simulink model "EMC_no_hand"  (R2015a)
settings: Solver=ode4  SolverMode=MultiTasking  StartTime=0.0  StopTime=inf  FixedStep=BKIN_STEP_TIME  RelTol=1e-3
StartFcn:
  |  warndlg('Dexterit-E models cannot run under simulation. Please compile your model and run it from within Dexterit-E.');set_param(bdroot,'SimulationCommand','stop')
model workspace (MAT data in the model file):
  BKIN_KINEMATIC_FRAME_SIZE = 400
  BKIN_STEP_TIME = 0.00025
  COLOR = 4
  COL_X = 1
  COL_Y = 2
  E_NO_EVENT = 0
  LOAD_X = 1
  LOAD_Y = 2
  MOVEMENT_DELAY = 3
  PATH_LENGTH = 1
  PATH_PERIOD = 2
  POST_TRIAL_DELAY = 4
  RADIUS = 3
  TRAJECTORY = 1
  TRAJECTORY_TYPE = 2
  TRIAL_END = 3
  TRIAL_MOVEMENT = 2
  TRIAL_RESET = 4
  TRIAL_START = 1
  X_POSITION = 1
  Y_POSITION = 2
  col_x = 1
  col_y = 2
  ANGULAR_THRESHOLD = 5
  GAZE_EXIT = 6
  START_REACHED = 7
  FIXATION_DURATION = 6
  TRACKING_TARGET_ROW = 7
  FEEDBACK_COLOR = 5
  CROSS_LOGICAL_RADIUS = 8
  DETECT_FIXATION = 8
  GAZE_IN_TARGET = 5
  START_STABILIZATION = 9
  HAND_IN_TARGET = 9
  BACKGROUND_LOAD = 10
  DIST_BETWEEN_TRAJ = 11
  STRAIGHT_PAUSE_TIME = 12
libraries: simulink x14, xpcrtudplib x12, xpcutilitieslib x10, xpcobsoletelib x8, slrtlib x2, ethercat x2, General x2, Video x2
(part 6 of 6)

== matlab function EMC_no_hand/DataLogging/Poll KINARM/createKINData/record errors ==
  data: newMessage output; ECATMessages input; cycle input; step_time input; sentMessageCount output
function [newMessage, sentMessageCount] = fcn(ECATMessages, cycle, step_time)

    persistent lastECATMessages outCount memoryBuffer waitingMsgCount sentCount
    
    if isempty(lastECATMessages)
        lastECATMessages = ECATMessages;
        memoryBuffer = zeros(50, 6);
        waitingMsgCount = 0;
        outCount = 0;
        sentCount = 0;
    end
    
    stepsPerFrame = 0.001 / step_time;

    %copy over the errors from ethercat drives
    for drive=1:4
        if waitingMsgCount >= 50
            continue;
        end
        
        if ECATMessages(drive, 3) ~= lastECATMessages(drive, 3) && ECATMessages(drive, 3) ~= 0
            waitingMsgCount = waitingMsgCount + 1;
%            memoryBuffer(waitingMsgCount,:) = [cycle, ECATMessages(drive,1), ECATMessages(drive,2), ECATMessages(drive,3), ECATMessages(drive, 4), ECATMessages(drive,5)];
            memoryBuffer(waitingMsgCount,1) = cycle;
            memoryBuffer(waitingMsgCount,2:6) = ECATMessages(drive,:);
        end
    end
    
    newMessage = zeros(1,6);
    %if we have an error to send we must send it for a few frames because we only send
    %some frames to the GUI computer. The only safe way to handle this is to count
    %the number of real-time frames vs the frequency we send to the GUI computer on.
    %I wanted to use the actual frame number we send to the GUI, but the trouble is
    %we don't know which of the kinematic frames gets sent to the GUI, it's just one
    %of the 2 or 4 that happens for each frame we send to the GUI. 
    %So instead here I cop out and just count 2 or 4 frames and then send something new.
    if waitingMsgCount > 0
        newMessage = memoryBuffer(1,:);
        outCount = outCount + 1;
        
        %we've sent the frame enough times...
        if outCount >= stepsPerFrame
            %shift the list so the first row is the next thing to send.
            memoryBuffer(1:end-1,:) = memoryBuffer(2:end,:);
            waitingMsgCount = waitingMsgCount - 1;
            sentCount = sentCount + 1;
            outCount = 0;  
            
            %if we still have another frame to send then copy it out..
            if waitingMsgCount > 0
                newMessage = memoryBuffer(1,:);
                outCount = 1;
            end
        end
    end
    
    lastECATMessages = ECATMessages;
    sentMessageCount = sentCount;
end

== matlab function EMC_no_hand/DataLogging/Poll KINARM/make KINData bus/splitKINData arm1 ==
  data: robot_row input; link_lengths output; pointer_offset output; shoulder_loc output; arm_orientation output; shoulder_ang output; elbow_ang output; shoulder_ang_velocity output; elbow_ang_velocity output; shoulder_ang_acceleration output; elbow_ang_acceleration output; joint_torque_cmd output; motor_torque_cmd output; link_angle output; link_velocity output; link_acceleration output; hand_position output; hand_velocity output; hand_acceleration output; elbow_position output; elbow_velocity output; elbow_acceleration output; motor_status output; force_sensor_force_uvw output; force_sensor_torque_uvw output; force_sensor_force_xyz output; force_sensor_torque_xyz output; force_sensor_timestamp output
function [link_lengths, pointer_offset, shoulder_loc, arm_orientation, ...
    shoulder_ang, elbow_ang, shoulder_ang_velocity, elbow_ang_velocity, shoulder_ang_acceleration, elbow_ang_acceleration, ...
    joint_torque_cmd, motor_torque_cmd, ...
    link_angle, link_velocity, link_acceleration, ...
    hand_position, hand_velocity, hand_acceleration, ...
    elbow_position, elbow_velocity, elbow_acceleration, ...
    motor_status, ...
    force_sensor_force_uvw, force_sensor_torque_uvw, force_sensor_force_xyz, force_sensor_torque_xyz, force_sensor_timestamp] = splitKINData(robot_row)

link_lengths = robot_row(1,1:2);                % L1, L2 length in m
pointer_offset = robot_row(1,3);                % perpendicular distance from L2 to subject pointer (m)
shoulder_loc = robot_row(1,4:5);                % shoulder x,y position (m) (global coordinates)
arm_orientation = robot_row(1,6);                % subject's expected arm orientation (1: right, 2: left)
shoulder_ang = robot_row(1,7);				% shoulder joint angle, with correction for offsets (see above) (rad)
elbow_ang = robot_row(1,8);					% elbow joint angle, with correction for offsets (see above) (rad)
shoulder_ang_velocity = robot_row(1,9);             % shoulder joint angular velocity (rad/s)
elbow_ang_velocity = robot_row(1,10);               % elbow joint angular velocity (rad/s)
shoulder_ang_acceleration = robot_row(1,11);        % shoulder joint angular acceleration (rad/s^2)
elbow_ang_acceleration = robot_row(1,12);           % elbow joint angular acceleration (rad/s^2)
joint_torque_cmd = robot_row(1,13:14);          % commanded shoulder (1), and elbow (2) torque (Nm)
motor_torque_cmd = robot_row(1,15:16);          % commanded motor 1 (1) and 2 (2) torque (shoulder torque less elbow torque) (Nm)

link_angle = robot_row(1,17:18);                % upper arm angle with corrections, orientation-independent (see above) (rad)
link_velocity = robot_row(1,19:20);             % upper arm angular velocity, orientation-independent (see above) (rad/s)
link_acceleration = robot_row(1,21:22);         % upper arm angular acceleration, orientation-independent (see above) (rad/s^2)


hand_position = robot_row(1,23:24);             % fingertip position in x,y (m)
hand_velocity = robot_row(1,25:26);             % fingertip velocity in x,y (m/s)
hand_acceleration = robot_row(1,27:28);         % fingertip acceleration in x,y (m/s^2)

elbow_position = robot_row(1,29:30);
elbow_velocity =  robot_row(1,31:32);
elbow_acceleration = robot_row(1,33:34);

% shoulder_velocity_filt = robot_row(1,35);
% elbow_velocity_filt = robot_row(1,36);

motor_status = robot_row(1,37);                 % motor status (bitfield; each 0: motor enabled, 1: motor disabled/faulted)

force_sensor_force_uvw = robot_row(1,38:40);    % force measured by force sensor along u,v,w in its local coordinate system (N)
force_sensor_torque_uvw = robot_row(1,41:43);   % torque measured by force sensor along u,v,w in its local coordinate system (Nm)

force_sensor_force_xyz = robot_row(1,44:46);    % force measured by force sensor along x,y,z in the global coordinate system (N)
force_sensor_torque_xyz = robot_row(1,47:49);   % torque measured by force sensor along x in its local coordinate system (Nm)
force_sensor_timestamp = robot_row(1,50);       % The timestamp from the force sensor(s)

end

== matlab function EMC_no_hand/DataLogging/Poll KINARM/make KINData bus/splitKINData arm2 ==
  data: robot_row input; link_lengths output; pointer_offset output; shoulder_loc output; arm_orientation output; shoulder_ang output; elbow_ang output; shoulder_ang_velocity output; elbow_ang_velocity output; shoulder_ang_acceleration output; elbow_ang_acceleration output; joint_torque_cmd output; motor_torque_cmd output; link_angle output; link_velocity output; link_acceleration output; hand_position output; hand_velocity output; hand_acceleration output; elbow_position output; elbow_velocity output; elbow_acceleration output; motor_status output; force_sensor_force_uvw output; force_sensor_torque_uvw output; force_sensor_force_xyz output; force_sensor_torque_xyz output; force_sensor_timestamp output
function [link_lengths, pointer_offset, shoulder_loc, arm_orientation, ...
    shoulder_ang, elbow_ang, shoulder_ang_velocity, elbow_ang_velocity, shoulder_ang_acceleration, elbow_ang_acceleration, ...
    joint_torque_cmd, motor_torque_cmd, ...
    link_angle, link_velocity, link_acceleration, ...
    hand_position, hand_velocity, hand_acceleration, ...
    elbow_position, elbow_velocity, elbow_acceleration, ...
    motor_status, ...
    force_sensor_force_uvw, force_sensor_torque_uvw, force_sensor_force_xyz, force_sensor_torque_xyz, force_sensor_timestamp] = splitKINData(robot_row)

link_lengths = robot_row(1,1:2);                % L1, L2 length in m
pointer_offset = robot_row(1,3);                % perpendicular distance from L2 to subject pointer (m)
shoulder_loc = robot_row(1,4:5);                % shoulder x,y position (m) (global coordinates)
arm_orientation = robot_row(1,6);                % subject's expected arm orientation (1: right, 2: left)
shoulder_ang = robot_row(1,7);				% shoulder joint angle, with correction for offsets (see above) (rad)
elbow_ang = robot_row(1,8);					% elbow joint angle, with correction for offsets (see above) (rad)
shoulder_ang_velocity = robot_row(1,9);             % shoulder joint angular velocity (rad/s)
elbow_ang_velocity = robot_row(1,10);               % elbow joint angular velocity (rad/s)
shoulder_ang_acceleration = robot_row(1,11);        % shoulder joint angular acceleration (rad/s^2)
elbow_ang_acceleration = robot_row(1,12);           % elbow joint angular acceleration (rad/s^2)
joint_torque_cmd = robot_row(1,13:14);          % commanded shoulder (1), and elbow (2) torque (Nm)
motor_torque_cmd = robot_row(1,15:16);          % commanded motor 1 (1) and 2 (2) torque (shoulder torque less elbow torque) (Nm)

link_angle = robot_row(1,17:18);                % upper arm angle with corrections, orientation-independent (see above) (rad)
link_velocity = robot_row(1,19:20);             % upper arm angular velocity, orientation-independent (see above) (rad/s)
link_acceleration = robot_row(1,21:22);         % upper arm angular acceleration, orientation-independent (see above) (rad/s^2)


hand_position = robot_row(1,23:24);             % fingertip position in x,y (m)
hand_velocity = robot_row(1,25:26);             % fingertip velocity in x,y (m/s)
hand_acceleration = robot_row(1,27:28);         % fingertip acceleration in x,y (m/s^2)

elbow_position = robot_row(1,29:30);
elbow_velocity =  robot_row(1,31:32);
elbow_acceleration = robot_row(1,33:34);

% shoulder_velocity_filt = robot_row(1,35);
% elbow_velocity_filt = robot_row(1,36);

motor_status = robot_row(1,37);                 % motor status (bitfield; each 0: motor enabled, 1: motor disabled/faulted)

force_sensor_force_uvw = robot_row(1,38:40);    % force measured by force sensor along u,v,w in its local coordinate system (N)
force_sensor_torque_uvw = robot_row(1,41:43);   % torque measured by force sensor along u,v,w in its local coordinate system (Nm)

force_sensor_force_xyz = robot_row(1,44:46);    % force measured by force sensor along x,y,z in the global coordinate system (N)
force_sensor_torque_xyz = robot_row(1,47:49);   % torque measured by force sensor along x in its local coordinate system (Nm)
force_sensor_timestamp = robot_row(1,50);       % The timestamp from the force sensor(s)

end

== matlab function EMC_no_hand/DataLogging/Poll KINARM/make KINData bus/splitKINDataGeneral ==
  data: kinarm_data input; active_arm output; delayEstimates output; servoCounter output; calibrationButtonBits output; robot_arm output; subject_arm output; handFF output; handFF_Dex output; handFBArm output; handFBRadius output; handFBControl output; handFBColor output; hasGaze output; gazeFB output; gazeLocation output; gazeTimestamp output; gazePupilArea output; gazeEvent output; gazeVector output; gazePupilLoc output; subject_arm_in input
function [active_arm, delayEstimates, servoCounter, calibrationButtonBits, robot_arm, subject_arm, ...
    handFF, handFF_Dex, handFBArm, handFBRadius, handFBControl, handFBColor, hasGaze, gazeFB, ...
    gazeLocation, gazeTimestamp, gazePupilArea, gazeEvent, gazeVector, gazePupilLoc] = splitKINData(kinarm_data, subject_arm_in)

    active_arm = kinarm_data(1);          % dominant KINARM for the experiment (1: arm 1, 2: arm 2)
    robot_arm = active_arm;               % trying to make a clearer named signal for what this really is
    subject_arm = subject_arm_in;         % I only do this so that the value can be sent to a scope!
    handFF = kinarm_data(2);              % duration of feed forward for position of hand feedback (s)
    handFF_Dex = kinarm_data(7);           % the true feed forward time set in Dexterit-E
    handFBArm = kinarm_data(3);           % hand feedback arm (0: none, 1: dominant, 2: non-dominant, 3: both, 4: controlled by task program)
    handFBControl = kinarm_data(4);       % hand feedback settings source (0: GUI, 1: from task program)
    handFBColor = kinarm_data(5);         % feedback colour (RRRGGGBBB string converted to integer)
    handFBRadius = kinarm_data(6);        % feedback radius (m)

    delayEstimates = kinarm_data(8:11);   % primary encoders velocity(1), acceleration(2), seconadary enc velocity(3) and acceleration(4) delay estimate (s)
    servoCounter = kinarm_data(12);       % servo update count
    calibrationButtonBits = kinarm_data(13);  % EP calibration button status bitfield


    hasGaze = kinarm_data(14);            % is Gaze tracking hardware available
    gazeFB = kinarm_data(15);             % Gaze feedback (0: on, 1: controlled by task program)

    gazeLocation = kinarm_data(16:17);    % Gaze X,Y location in global coordinates
    gazeTimestamp = kinarm_data(18);      % Gaze Timestamp in seconds
    gazePupilArea = kinarm_data(19);      % Gaze pupil area
    gazeEvent = kinarm_data(20:22);       % Gaze Event ID(1), start time(2), end time (3) 
    gazeVector = kinarm_data(23:25);      % Gaze vector in global coordinates
    gazePupilLoc = kinarm_data(26:28);    % Gaze pupil location in global coordinates
end

== matlab function EMC_no_hand/DataLogging/Poll KINARM/split_primary/split_primary ==
  data: primary_data input; link_angles output; link_velocities output; link_acceleration output
function [link_angles, link_velocities, link_acceleration] = splitPrimary(primary_data)
   link_angles = primary_data(1:2);
   link_velocities = primary_data(3:4);
   link_acceleration = primary_data(5:6);
end

== matlab function EMC_no_hand/DataLogging/Poll KINARM/split_primary/split_primary1 ==
  data: primary_data input; link_angles output; link_velocities output; link_acceleration output
function [link_angles, link_velocities, link_acceleration] = splitPrimary(primary_data)
   link_angles = primary_data(1:2);
   link_velocities = primary_data(3:4);
   link_acceleration = primary_data(5:6);
end

== matlab function EMC_no_hand/DataLogging/apply loads/verify NaN ==
  data: torques_in input; torques_out output
function torques_out  = fcn(torques_in)
%#codegen

persistent check isWorking

if isempty(check)
    check = 1;

    % The code generator tries to be very smart when converting this to C.
    % if you do something simple like isinf(inf) or isnan(nan) then those
    % statements are optimized out of the C for always being true. The code
    % below is an attempt to outsmart the converted to actually generate
    % real C code that should generate nan or inf. From what I can tell,
    % at least in R2018a this gets generated to proper code that does these
    % checks the way I want.
    
    sq = rand();
    while sq > 0.99
        sq = rand();
    end
    
    r = ceil(rand());
    mr = -r;
    r = r * 2;
    
    % DEX-3729, DEX-3732
    % if the wrong compiler options are used then "fast math" could be
    % enabled. Fast math breaks checks for NaN. If we can't tell if a number
    % is NaN then we need to force all output forces to zero.
    % it appears that checking for inf always works, but checking for
    % isfinite is broken with isnan.
    if ~isnan(sqrt(sq - 0.99)) || ~isinf(1.0 / (r + mr + mr))
        isWorking = 0;
        fprintf('***WARNING****');
        fprintf('Checks for NaN/inf FAIL. No forces will be produced.\n')
    else
        isWorking = 1;
        fprintf('Checks for NaN/inf WORK.\n')
    end
    
end

torques_out = torques_in;

% DEX-3729, DEX-3732
% if the wrong compiler options are used then "fast math" could be
% enabled. Fast math breaks checks for NaN. If we can't tell if a number
% is NaN then we need to force all output forces to zero.
if isWorking
    if sum(isnan(torques_out)) > 0
        torques_out(isnan(torques_out)) = 0;
    end
    
    if sum(isinf(torques_out)) > 0
        torques_out(isinf(torques_out)) = 0;
    end
else
    torques_out(:) = 0;
end

== matlab function EMC_no_hand/DataLogging/compare encoders/delta ==
  data: secondaryEncAngles input; deltas output; primaryEncAngles input
function deltas = fcn(secondaryEncAngles, primaryEncAngles)
%#eml

deltas = secondaryEncAngles - primaryEncAngles;

== matlab function EMC_no_hand/DataLogging/create_lab_info/Subsystem/MATLAB Function ==
  data: orientation input; is_right_arm output; has_secondary input; isEP input; isExo output; has_high_res_encoders output
function [is_right_arm, isExo, has_high_res_encoders] = fcn(orientation, has_secondary, isEP)
%#codegen

isExo = 1;
if isEP
    isExo = 0;
end

has_high_res_encoders = has_secondary;

is_right_arm = 0;
if (isExo && orientation == 1) || (isEP && orientation == -1)
    is_right_arm = 1;
end

== matlab function EMC_no_hand/DataLogging/create_lab_info/Subsystem/MATLAB Function1 ==
  data: orientation input; is_right_arm output; has_secondary input; isEP input; isExo output; has_high_res_encoders output
function [is_right_arm, isExo, has_high_res_encoders] = fcn(orientation, has_secondary, isEP)
%#codegen

isExo = 1;
if isEP
    isExo = 0;
end

has_high_res_encoders = has_secondary;

is_right_arm = 0;
if (isExo && orientation == 1) || (isEP && orientation == -1)
    is_right_arm = 1;
end

== matlab function EMC_no_hand/DataLogging/monitor torques/MATLAB Function ==
  data: robot_failures output; torque_err_bitfield output; cmd input; abs_diff output; rec input; threshold_rel_diff input; rel_diff output; threshold_abs_diff input
function [robot_failures, torque_err_bitfield, abs_diff, rel_diff] = fcn(cmd, rec, threshold_rel_diff, threshold_abs_diff)
%#codegen

abs_diff = abs(cmd - rec);
rel_diff = abs_diff ./ cmd;
rel_diff(~isfinite(rel_diff)) = 0;

out_of_spec_motors = (abs_diff >= threshold_abs_diff) + (rel_diff >= threshold_rel_diff);
robot_failures = [sum(out_of_spec_motors(1:2) == 2) > 0, sum(out_of_spec_motors(3:4) == 2) > 0];
torque_errors = out_of_spec_motors == 2;
torque_err_bitfield = sum(bitshift(uint32(torque_errors'), 0:3));

== stateflow chart EMC_no_hand/DataLogging/monitor torques/torque_monitor ==
  state init/
    command_multiplier = 1;
    stop_vel_mode = 0;
    robot_err_bits_out = 0;
  state Done/
  state Monitoring/
  state EpMonitor/
    state Robot1/ [parallel]
      settings: executionOrder=1
      state not_holding/
      state Waiting/
      note: After the current limit stops we need
          | to wait a bit before currents are back to full force
      state CurrentLimited/
      state Pause/
      state Err/
        command_multiplier = 0;
        stop_vel_mode = 1;
      (default) -> EpMonitor.Robot1.Waiting
      EpMonitor.Robot1.Waiting -> EpMonitor.Robot1.not_holding [order 1] : [e_grips[1] == 0 || robot_scaling[1] != 1]
      EpMonitor.Robot1.not_holding -> EpMonitor.Robot1.Waiting : [e_grips[1] == 1 && robot_scaling[1] == 1]
      EpMonitor.Robot1.Waiting -> (junction 47) [order 2]
      EpMonitor.Robot1.Pause -> EpMonitor.Robot1.not_holding : after(1000, e_clk)
      EpMonitor.Robot1.CurrentLimited -> EpMonitor.Robot1.Pause : [current_limit_enabled[1] == 0]
      (junction 47) -> EpMonitor.Robot1.CurrentLimited [order 1] : [current_limit_enabled[1] != 0]
      (junction 47) -> EpMonitor.Robot1.Err [order 2] : [robot_error[1] == 1]
          | {robot_err_bits_out = robot_err_bits_in;}
    state Robot2/ [parallel]
      settings: executionOrder=2
      state not_holding/
      state Waiting/
      state CurrentLimited/
      state Pause/
      state Err/
        command_multiplier = 0;
        stop_vel_mode = 1;
      (default) -> EpMonitor.Robot2.Waiting
      EpMonitor.Robot2.Waiting -> EpMonitor.Robot2.not_holding [order 1] : [e_grips[2] == 0 || robot_scaling[2] != 1]
      EpMonitor.Robot2.not_holding -> EpMonitor.Robot2.Waiting : [e_grips[2] == 1 && robot_scaling[2] == 1]
      EpMonitor.Robot2.Waiting -> (junction 68) [order 2]
      EpMonitor.Robot2.Pause -> EpMonitor.Robot2.not_holding : after(1000, e_clk)
      EpMonitor.Robot2.CurrentLimited -> EpMonitor.Robot2.Pause : [current_limit_enabled[2] == 0]
      (junction 68) -> EpMonitor.Robot2.CurrentLimited [order 1] : [current_limit_enabled[2] != 0]
      (junction 68) -> EpMonitor.Robot2.Err [order 2] : [robot_error[2] == 1]
          | {robot_err_bits_out = robot_err_bits_in;}
  state ExoMonitor/
  state eStopdown/
  state Wait/
  state CurrentLimited/
  state ErrorFound/
    command_multiplier = 0;
  (default) -> init
  init -> Done [order 1] : [is_ecat == 0]
  init -> Monitoring [order 2] : after(2000, e_clk)
  Monitoring -> EpMonitor [order 1] : [is_ep == 1]
  Monitoring -> ExoMonitor [order 2]
  ExoMonitor -> eStopdown [order 1] : [robot_scaling[1] != 1 || robot_scaling[2] != 1]
  eStopdown -> ExoMonitor : [robot_scaling[1] == 1 && robot_scaling[2] == 1]
  Wait -> eStopdown : after(1000, e_clk)
  ExoMonitor -> (junction 80) [order 2]
  (junction 84) -> Wait
  CurrentLimited -> (junction 84) : [current_limit_enabled[3] == 0]
  (junction 80) -> CurrentLimited [order 2] : [current_limit_enabled[3] != 0]
  (junction 80) -> ErrorFound [order 1] : [robot_error[1] == 1 || robot_error[2] == 1]
      | {robot_err_bits_out = robot_err_bits_in;}
  data: e_grips input size=2; robot_scaling input double size=2; current_limit_enabled input double size=3; command_multiplier output double size=1; is_ep input double; is_ecat input boolean; robot_error input size=2; stop_vel_mode output double; robot_err_bits_in input double; robot_err_bits_out output double
  events: e_clk input RISING_EDGE_EVENT
